simulink model "uavCtrl"  (R2024b)
settings: Solver=VariableStepAuto  StartTime=0.0  StopTime=10.0  RelTol=1e-3
settings Model: Creator=win10-s  LastModifiedBy=rzxha
settings SolverCC: AlgebraicLoopSolver=TrustRegion
settings DataIOCC: ReturnWorkspaceOutputs=off
settings DebuggingCC: UnconnectedInputMsg=warning  UnconnectedOutputMsg=warning  UnconnectedLineMsg=warning  ArithmeticOperatorsInVariantConditions=warning
settings ModelReferenceCC: EnableRefExpFcnMdlSchedulingChecks=on
settings SFSimCC: CustomCodeUndefinedFunction=UseInterfaceOnly
settings RTWCC: GPUComputeCapability=3.5

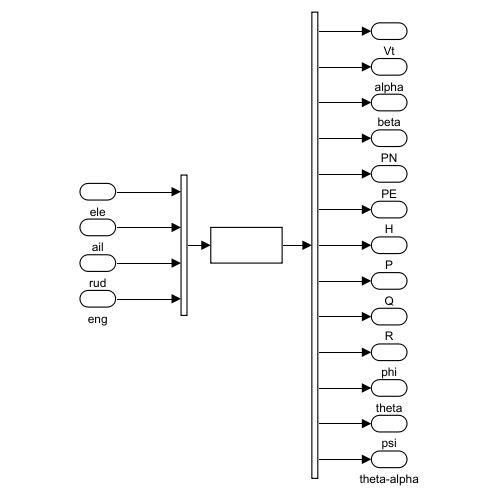
[thumbnail: Simulink's stored preview of the top-level diagram]
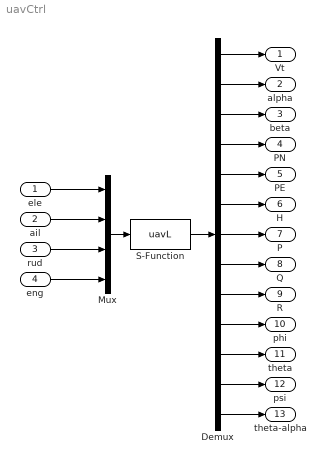
== system uavCtrl ==
  ele : Inport
  ail : Inport  Port=2
  rud : Inport  Port=3
  eng : Inport  Port=4
  Demux : Demux  Outputs=13
  Mux : Mux
  S-Function : S-Function  FunctionName=uavL  SFunctionDeploymentMode=off  EnableBusSupport=off
  Vt : Outport  VectorParamsAs1DForOutWhenUnconnected=off
  alpha : Outport  Port=2  VectorParamsAs1DForOutWhenUnconnected=off
  beta : Outport  Port=3  VectorParamsAs1DForOutWhenUnconnected=off
  PN : Outport  Port=4  VectorParamsAs1DForOutWhenUnconnected=off
  PE : Outport  Port=5  VectorParamsAs1DForOutWhenUnconnected=off
  H : Outport  Port=6  VectorParamsAs1DForOutWhenUnconnected=off
  P : Outport  Port=7  VectorParamsAs1DForOutWhenUnconnected=off
  Q : Outport  Port=8  VectorParamsAs1DForOutWhenUnconnected=off
  R : Outport  Port=9  VectorParamsAs1DForOutWhenUnconnected=off
  phi : Outport  Port=10  VectorParamsAs1DForOutWhenUnconnected=off
  theta : Outport  Port=11  VectorParamsAs1DForOutWhenUnconnected=off
  psi : Outport  Port=12  VectorParamsAs1DForOutWhenUnconnected=off
  theta-alpha : Outport  Port=13  VectorParamsAs1DForOutWhenUnconnected=off
  wires:
  Mux/1 -> S-Function/1
  ele/1 -> Mux/1
  ail/1 -> Mux/2
  rud/1 -> Mux/3
  eng/1 -> Mux/4
  S-Function/1 -> Demux/1
  Demux/1 -> Vt/1
  Demux/2 -> alpha/1
  Demux/3 -> beta/1
  Demux/4 -> PN/1
  Demux/8 -> Q/1
  Demux/7 -> P/1
  Demux/6 -> H/1
  Demux/5 -> PE/1
  Demux/9 -> R/1
  Demux/10 -> phi/1
  Demux/11 -> theta/1
  Demux/12 -> psi/1
  Demux/13 -> theta-alpha/1
